simulink model "FLC_PID_Robot_Control_Full"  (R2020b)
settings: Solver=ode4  StartTime=0.0  StopTime=50  FixedStep=0.01  RelTol=1e-3
values from neighbouring files (symbols this model uses):
  a = 0    [Robot_Parameters.m]
  b = 0.2    [Robot_Parameters.m]
  I = 0.08    [Robot_Parameters.m]
  Ke = 0.03    [Robot_Parameters.m]
  Kt = 0.001    [Robot_Parameters.m]
  L = 0.01    [Robot_Parameters.m]
  m = 1.733    [Robot_Parameters.m]
  N = 30    [Robot_Parameters.m]
  r = 0.0425    [Robot_Parameters.m]
  R = 0.7    [Robot_Parameters.m]
libraries: pid_lib x2, fuzblock x1, mobileRoboticsLib x1, simulink x1
settings Model: OrderedModelArguments=off  Creator=dell  LastModifiedBy=dell

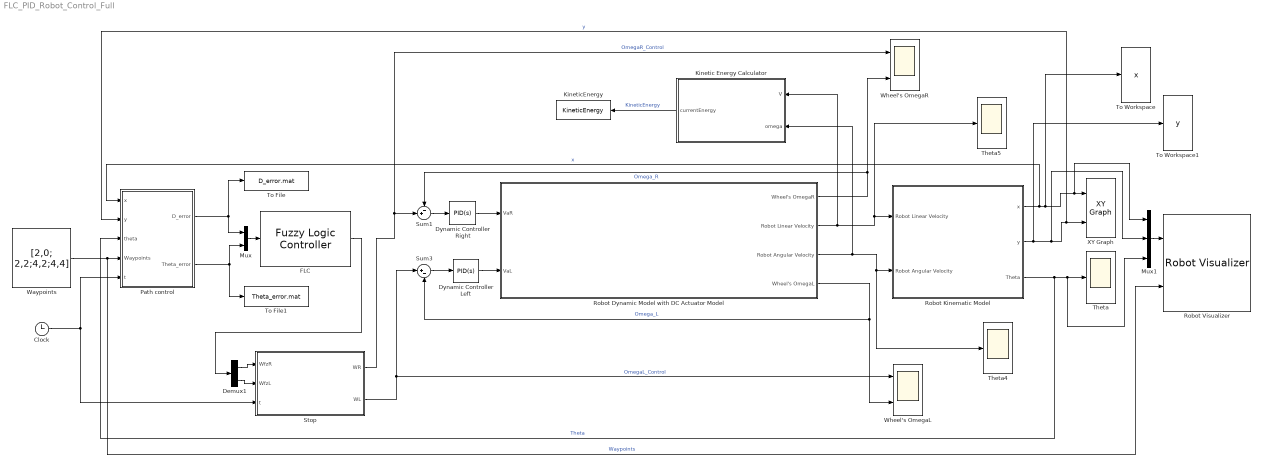
== system FLC_PID_Robot_Control_Full ==
  Clock : Clock
  Demux1 : Demux  Outputs=2
  Dynamic Controller Left : pid_lib/PID Controller  Controller=PID  Form=Parallel  TimeDomain=Continuous-time  UseExternalTs=off  SampleTime=-1  IntegratorMethod=Forward Euler  FilterMethod=Forward Euler  ControllerParametersSource=internal  P=0.75291038869307  I=8.52783510111841  D=-0.0138279489870919  UseFilter=on  N=14.2847240550013  TunerSelectOption=Transfer Function Based (PID Tuner App)  InitialConditionSource=internal  InitialConditionForIntegrator=0  InitialConditionForFilter=0  DifferentiatorICPrevScaledInput=0  ExternalReset=none  TrackingMode=off  Kt=1  LimitOutput=off  SatLimitsSource=internal  UpperSaturationLimit=inf  LowerSaturationLimit=-inf  LinearizeAsGain=on  AntiWindupMode=none  Kb=1  POutMin=[]  POutMax=[]  IOutMin=[]  IOutMax=[]  DOutMin=[]  DOutMax=[]  NOutMin=[]  NOutMax=[]  SumOutMin=[]  SumOutMax=[]  SaturationOutMin=[]  SaturationOutMax=[]  PParamMin=[]  PParamMax=[]  IParamMin=[]  IParamMax=[]  DParamMin=[]  DParamMax=[]  NParamMin=[]  NParamMax=[]  KbParamMin=[]  KbParamMax=[]  KtParamMin=[]  KtParamMax=[]  KbOutMin=[]  KbOutMax=[]  KtOutMin=[]  KtOutMax=[]  IntegratorOutMin=[]  IntegratorOutMax=[]  FilterOutMin=[]  FilterOutMax=[]  SumI1OutMin=[]  SumI1OutMax=[]  SumI2OutMin=[]  SumI2OutMax=[]  SumI3OutMin=[]  SumI3OutMax=[]  SumI4OutMin=[]  SumI4OutMax=[]  SumDOutMin=[]  SumDOutMax=[]  DifferentiatorOutMin=[]  DifferentiatorOutMax=[]  FilterDiffOutCoefMin=[]  FilterDiffOutCoefMax=[]  ReciprocalOutMin=[]  ReciprocalOutMax=[]  SumDenOutMin=[]  SumDenOutMax=[]  SumNumOutMin=[]  SumNumOutMax=[]  DivideOutMin=[]  DivideOutMax=[]  UdiffTsProdOutMin=[]  UdiffTsProdOutMax=[]  NTsProdOutMin=[]  NTsProdOutMax=[]  UintegralTsProdOutMin=[]  UintegralTsProdOutMax=[]  UngainTsProdOutMin=[]  UngainTsProdOutMax=[]  IntegratorContinuousStateAttributes=''  IntegratorStateMustResolveToSignalObject=off  IntegratorRTWStateStorageClass=Auto  FilterContinuousStateAttributes=''  FilterStateMustResolveToSignalObject=off  FilterRTWStateStorageClass=Auto  ParallelPVariant=InternalParameters  IdealPVariant=Disabled  IVariant=InternalParameters  DVariant=InternalParameters  IntegratorVariant=Continuous  SatVariant=Disabled  AWVariant=Passthrough  PCopyVariant=Disabled  TRVariant=Disabled  FdbkBlocksVariant=Forward  IdealPFdbkVariant=Disabled  SatFdbkVariant=Disabled  DerivativeFilterVariant=ContFilter  NVariant=InternalParameters  NCopyVariant=Disabled  FilterICVariant=InternalICsFilter  IntegratorICVariant=InternalICs  ExternalResetVariant=Disabled  TRSumVariant=Passthrough  SumFdbkVariant=Disabled  SumVariant=Sum_PID  TsampFilterVariant=InternalTs  TsampNgainVariant=Passthrough  TsampIntegralVariant=Passthrough  ExternalSaturationOutDataTypeStr=Inherit: Same as second input
  Dynamic Controller Right : pid_lib/PID Controller  Controller=PID  Form=Parallel  TimeDomain=Continuous-time  UseExternalTs=off  SampleTime=-1  IntegratorMethod=Forward Euler  FilterMethod=Forward Euler  ControllerParametersSource=internal  P=0.926055377132756  I=9.27563715391367  D=-0.025  UseFilter=on  N=20.0890041410903  TunerSelectOption=Transfer Function Based (PID Tuner App)  ZeroCross=off  InitialConditionSource=internal  InitialConditionForIntegrator=0  InitialConditionForFilter=0  DifferentiatorICPrevScaledInput=0  ExternalReset=none  TrackingMode=off  Kt=1  LimitOutput=off  SatLimitsSource=internal  UpperSaturationLimit=inf  LowerSaturationLimit=-inf  LinearizeAsGain=on  AntiWindupMode=none  Kb=1  POutMin=[]  POutMax=[]  IOutMin=[]  IOutMax=[]  DOutMin=[]  DOutMax=[]  NOutMin=[]  NOutMax=[]  SumOutMin=[]  SumOutMax=[]  SaturationOutMin=[]  SaturationOutMax=[]  PParamMin=[]  PParamMax=[]  IParamMin=[]  IParamMax=[]  DParamMin=[]  DParamMax=[]  NParamMin=[]  NParamMax=[]  KbParamMin=[]  KbParamMax=[]  KtParamMin=[]  KtParamMax=[]  KbOutMin=[]  KbOutMax=[]  KtOutMin=[]  KtOutMax=[]  IntegratorOutMin=[]  IntegratorOutMax=[]  FilterOutMin=[]  FilterOutMax=[]  SumI1OutMin=[]  SumI1OutMax=[]  SumI2OutMin=[]  SumI2OutMax=[]  SumI3OutMin=[]  SumI3OutMax=[]  SumI4OutMin=[]  SumI4OutMax=[]  SumDOutMin=[]  SumDOutMax=[]  DifferentiatorOutMin=[]  DifferentiatorOutMax=[]  FilterDiffOutCoefMin=[]  FilterDiffOutCoefMax=[]  ReciprocalOutMin=[]  ReciprocalOutMax=[]  SumDenOutMin=[]  SumDenOutMax=[]  SumNumOutMin=[]  SumNumOutMax=[]  DivideOutMin=[]  DivideOutMax=[]  UdiffTsProdOutMin=[]  UdiffTsProdOutMax=[]  NTsProdOutMin=[]  NTsProdOutMax=[]  UintegralTsProdOutMin=[]  UintegralTsProdOutMax=[]  UngainTsProdOutMin=[]  UngainTsProdOutMax=[]  IntegratorContinuousStateAttributes=''  IntegratorStateMustResolveToSignalObject=off  IntegratorRTWStateStorageClass=Auto  FilterContinuousStateAttributes=''  FilterStateMustResolveToSignalObject=off  FilterRTWStateStorageClass=Auto  ParallelPVariant=InternalParameters  IdealPVariant=Disabled  IVariant=InternalParameters  DVariant=InternalParameters  IntegratorVariant=Continuous  SatVariant=Disabled  AWVariant=Passthrough  PCopyVariant=Disabled  TRVariant=Disabled  FdbkBlocksVariant=Forward  IdealPFdbkVariant=Disabled  SatFdbkVariant=Disabled  DerivativeFilterVariant=ContFilter  NVariant=InternalParameters  NCopyVariant=Disabled  FilterICVariant=InternalICsFilter  IntegratorICVariant=InternalICs  ExternalResetVariant=Disabled  TRSumVariant=Passthrough  SumFdbkVariant=Disabled  SumVariant=Sum_PID  TsampFilterVariant=InternalTs  TsampNgainVariant=Passthrough  TsampIntegralVariant=Passthrough  ExternalSaturationOutDataTypeStr=Inherit: Same as second input
  FLC : fuzblock/Fuzzy Logic  Controller  FIS="\"D:\\PhDDATA\\PhDBrno\\Final_Dissertation\\Experiment\\SoftWare_Hardwares\\FLC_PID_Robot_Control_Full\\FuzzyLogicControllers_FIS\\Proposed_GA_FLC.fis\""  OutputSampleNumber=101  DataType=double  FuzzifiedInputs=off  RuleFiringStrengths=off  RuleOutputs=off  AggregatedOutputs=off  SimulateUsing=Interpreted execution  OutOfRangeInputValueMessage=warning  NoRuleFiredMessage=warning  EmptyOutputFuzzySetMessage=warning
  Kinetic Energy Calculator : MATLAB Function  TreatAsAtomicUnit=on
  KineticEnergy : ToWorkspace  VariableName=KineticEnergy  SaveFormat=Timeseries  SampleTime=-1
  Mux : Mux  Inputs=2
  Mux1 : Mux  Inputs=3
  Path control : MATLAB Function  TreatAsAtomicUnit=on
  Robot Dynamic Model with DC Actuator Model : Subsystem
  Robot Kinematic Model : Subsystem
  Robot Visualizer : mobileRoboticsLib/Environments/Robot Visualizer  Priority=99  robotRadius=0.0425  showTrajectory=on  hasWaypoints=on  hasLidar=off  sensorOffset=[ 0 0 ]  scanAngles=0  hasObjDetector=off  objDetectorOffset=[ 0, 0 ]  objDetectorAngle=0  objDetectorFOV=0  objDetectorMaxRange=0  objectColors=0  objectMarkers=s
      settings: SourceProductName=Ground Vehicles Library
  Stop : MATLAB Function  TreatAsAtomicUnit=on
  Sum1 : Sum  Inputs=-+|
  Sum3 : Sum  Inputs=|+-
  Theta : Scope
  Theta4 : Scope
  Theta5 : Scope
  To File : ToFile  Filename=D_error.mat  SaveFormat=Timeseries
  To File1 : ToFile  Filename=Theta_error.mat  SaveFormat=Timeseries
  To Workspace : ToWorkspace  VariableName=x  SaveFormat=Timeseries  SampleTime=-1
  To Workspace1 : ToWorkspace  VariableName=y  SaveFormat=Timeseries  SampleTime=-1
  Waypoints : Constant  Value=[2,0; 2,2;4,2;4,4]  SampleTime=-1
  Wheel's OmegaL : Scope  NumInputPorts=2
  Wheel's OmegaR : Scope  NumInputPorts=2
  XY Graph : simulink/Sinks/XY Graph  xmin=-2.5  xmax=6  ymin=-0.5  ymax=6  st=-1
  wires:
  Sum1/1 -> Dynamic Controller Right/1
  Sum3/1 -> Dynamic Controller Left/1
  Robot Kinematic Model/1(x) -> To Workspace/1, XY Graph/1, Mux1/1, Path control/1(x)  "x"
  Robot Kinematic Model/2(y) -> To Workspace1/1, XY Graph/2, Path control/2(y), Mux1/2  "y"
  Robot Kinematic Model/3(Theta) -> Theta/1, Mux1/3, Path control/3(theta)  "Theta"
  Robot Dynamic Model with DC Actuator Model/2(Robot Linear Velocity) -> Robot Kinematic Model/1(Robot Linear Velocity), Theta5/1, Kinetic Energy Calculator/1(V)
  Dynamic Controller Right/1 -> Robot Dynamic Model with DC Actuator Model/1(VaR)
  Dynamic Controller Left/1 -> Robot Dynamic Model with DC Actuator Model/2(VaL)
  Robot Dynamic Model with DC Actuator Model/4(Wheel's OmegaL) -> Sum3/2, Wheel's OmegaL/2  "Omega_L"
  Stop/1(WR) -> Wheel's OmegaR/1, Sum1/2  "OmegaR_Control"
  Stop/2(WL) -> Sum3/1, Wheel's OmegaL/1  "OmegaL_Control"
  Mux/1 -> FLC/1
  Path control/1(D_error) -> Mux/1, To File/1
  Path control/2(Theta_error) -> Mux/2, To File1/1
  Waypoints/1 -> Robot Visualizer/2, Path control/4(Waypoints)  "Waypoints"
  Mux1/1 -> Robot Visualizer/1
  Robot Dynamic Model with DC Actuator Model/1(Wheel's OmegaR) -> Wheel's OmegaR/2, Sum1/1  "Omega_R"
  Kinetic Energy Calculator/1(currentEnergy) -> KineticEnergy/1  "KineticEnergy"
  Robot Dynamic Model with DC Actuator Model/3(Robot Angular Velocity) -> Robot Kinematic Model/2(Robot Angular Velocity), Theta4/1, Kinetic Energy Calculator/2(omega)
  Demux1/1 -> Stop/1(WfzR)
  Demux1/2 -> Stop/2(WfzL)
  FLC/1 -> Demux1/1
  Clock/1 -> Path control/5(t), Stop/3(t)

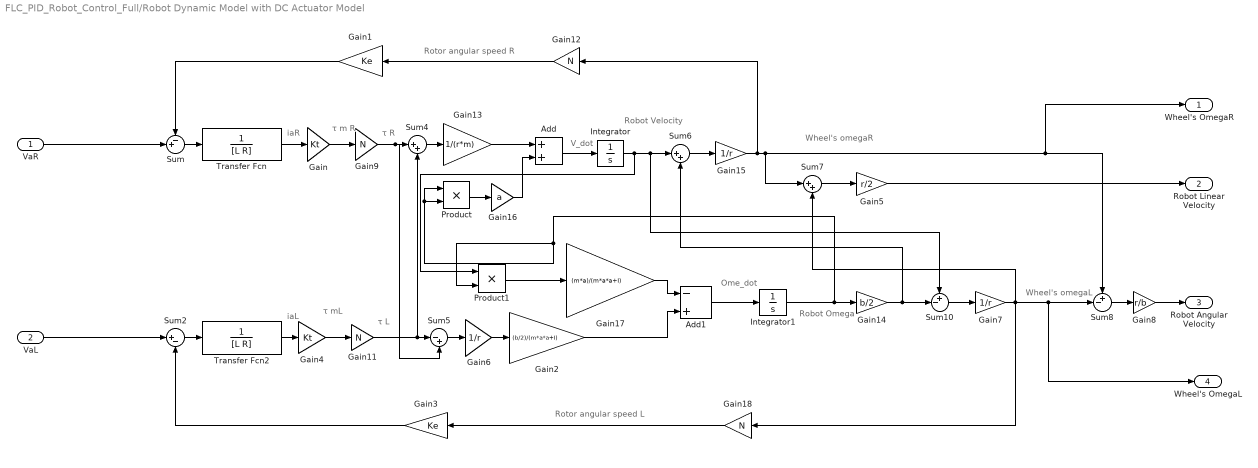
== system FLC_PID_Robot_Control_Full/Robot Dynamic Model with DC Actuator Model ==
  note: Rotor angular speed R
  note: Robot Velocity
  note: V_dot
  note: Robot Omega
  note: Ome_dot
  note: τ R
  note: τ m R
  note: iaR
  note: iaL
  note: τ mL
  note: τ L
  note: Rotor angular speed L
  note: Wheel's omegaR
  note: Wheel's omegaL
  VaR : Inport
  VaL : Inport  Port=2
  Add : Sum
  Add1 : Sum  Inputs=-+
  Gain : Gain  Gain=Kt
  Gain1 : Gain  Gain=Ke
  Gain{9,11..12,18} (4 alike) : Gain  Gain=N
  Gain13 : Gain  Gain=1/(r*m)
  Gain14 : Gain  Gain=b/2
  Gain15 : Gain  Gain=1/r
  Gain16 : Gain  Gain=a
  Gain17 : Gain  Gain=(m*a)/(m*a*a+I)
  Gain2 : Gain  Gain=(b/2)/(m*a*a+I)
  Gain3 : Gain  Gain=Ke
  Gain4 : Gain  Gain=Kt
  Gain5 : Gain  Gain=r/2
  Gain6 : Gain  Gain=1/r
  Gain7 : Gain  Gain=1/r
  Gain8 : Gain  Gain=r/b
  Integrator : Integrator
  Integrator1 : Integrator
  Product : Product
  Product1 : Product
  Sum : Sum  Inputs=-+|
  Sum10 : Sum  Inputs=+-|
  Sum2 : Sum  Inputs=|+-
  Sum4 : Sum  Inputs=|++
  Sum5 : Sum  Inputs=|-+
  Sum6 : Sum  Inputs=|++
  Sum7 : Sum  Inputs=|++
  Sum8 : Sum  Inputs=+-|
  Transfer Fcn : TransferFcn  Denominator=[L R]
  Transfer Fcn2 : TransferFcn  Denominator=[L R]
  Wheel's OmegaR : Outport
  Robot Linear Velocity : Outport  Port=2
  Robot Angular Velocity : Outport  Port=3
  Wheel's OmegaL : Outport  Port=4
  wires:
  Gain8/1 -> Robot Angular Velocity/1
  Gain5/1 -> Robot Linear Velocity/1
  Integrator/1 -> Sum6/1, Sum10/1, Product1/1
  Gain2/1 -> Add1/2
  Gain4/1 -> Gain11/1
  Sum6/1 -> Gain15/1
  Gain14/1 -> Sum10/2, Sum6/2
  Gain1/1 -> Sum/1
  Gain15/1 -> Gain12/1, Wheel's OmegaR/1, Sum8/1, Sum7/1
  Sum7/1 -> Gain5/1
  Gain6/1 -> Gain2/1
  Integrator1/1 -> Gain14/1, Product/2, Product/1, Product1/2
  Sum10/1 -> Gain7/1
  Product1/1 -> Gain17/1
  Transfer Fcn2/1 -> Gain4/1
  Sum/1 -> Transfer Fcn/1
  Gain17/1 -> Add1/1
  Add/1 -> Integrator/1
  Add1/1 -> Integrator1/1
  Gain12/1 -> Gain1/1
  Gain7/1 -> Wheel's OmegaL/1, Sum8/2, Sum7/2, Gain18/1
  Product/1 -> Gain16/1
  Gain9/1 -> Sum4/1, Sum5/2
  Gain/1 -> Gain9/1
  Gain11/1 -> Sum5/1, Sum4/2
  Gain16/1 -> Add/2
  Sum8/1 -> Gain8/1
  Gain18/1 -> Gain3/1
  Sum2/1 -> Transfer Fcn2/1
  Gain3/1 -> Sum2/2
  VaL/1 -> Sum2/1
  Transfer Fcn/1 -> Gain/1
  Gain13/1 -> Add/1
  Sum4/1 -> Gain13/1
  Sum5/1 -> Gain6/1
  VaR/1 -> Sum/2

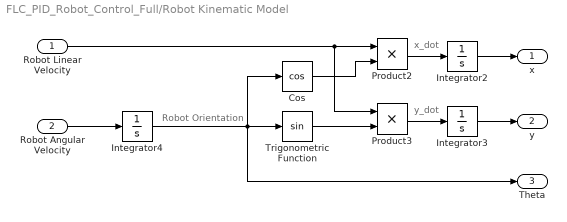
== system FLC_PID_Robot_Control_Full/Robot Kinematic Model ==
  note: x_dot
  note: Robot Orientation
  note: y_dot
  Robot Linear Velocity : Inport
  Robot Angular Velocity : Inport  Port=2
  Cos : Trigonometry  Operator=cos
  Integrator2 : Integrator
  Integrator3 : Integrator
  Integrator4 : Integrator
  Product2 : Product
  Product3 : Product
  Trigonometric Function : Trigonometry
  x : Outport
  y : Outport  Port=2
  Theta : Outport  Port=3
  wires:
  Trigonometric Function/1 -> Product3/2
  Cos/1 -> Product2/2
  Robot Linear Velocity/1 -> Product2/1, Product3/1
  Integrator4/1 -> Cos/1, Theta/1, Trigonometric Function/1
  Integrator2/1 -> x/1
  Product3/1 -> Integrator3/1
  Product2/1 -> Integrator2/1
  Integrator3/1 -> y/1
  Robot Angular Velocity/1 -> Integrator4/1

== matlab function FLC_PID_Robot_Control_Full/Path control ==
  data: x input; y input; theta input; D_error output; Theta_error output; Waypoints input; t input
%----------------------------------------------------------------------------------------------
%--------------------------------------------------------------------------------------------
function [D_error, Theta_error] = fcn(x,y,theta,Waypoints,t)
%  Go to the Waypoint 1
Pi = 3.14;
distanceEps = 0.01;
x_w = Waypoints(1,1);
y_w = Waypoints(1,2);
deltaX = x_w - x;
deltaY = y_w - y;
D_error = sqrt(deltaX^2 + deltaY^2);
Theta_w = atan2(deltaY,deltaX);
Theta_error = Theta_w - theta;
if Theta_error > Pi
    Theta_error = Theta_error - 2*Pi;
end
if Theta_error < -Pi
    Theta_error = Theta_error + 2*Pi;
end 
%  Go to the Waypoint 2
if D_error < distanceEps
    i = 2;
    x_w = Waypoints(i,1);
    y_w = Waypoints(i,2);
    deltaX = x_w - x;
    deltaY = y_w - y;
    D_error = sqrt(deltaX^2 + deltaY^2)
    Theta_w = atan2(deltaY,deltaX);
    Theta_error = Theta_w - theta;
    if Theta_error > Pi
        Theta_error = Theta_error- 2*Pi;
    end
    if Theta_error < -Pi
        Theta_error = Theta_error + 2*Pi;
    end
elseif (D_error >= distanceEps) && (t >= 5.31)
    i = 2;
    x_w = Waypoints(i,1);
    y_w = Waypoints(i,2);
    deltaX = x_w - x;
    deltaY = y_w - y;
    D_error = sqrt(deltaX^2 + deltaY^2)
    Theta_w = atan2(deltaY,deltaX);
    Theta_error = Theta_w - theta;
    if Theta_error > Pi
        Theta_error = Theta_error- 2*Pi;
    end
    if Theta_error < -Pi
        Theta_error = Theta_error + 2*Pi;
    end
    %  Go to the Waypoint 3
    if D_error < distanceEps
        i = 3;
        x_w = Waypoints(i,1);
        y_w = Waypoints(i,2);
        deltaX = x_w - x;
        deltaY = y_w - y;
        D_error = sqrt(deltaX^2 + deltaY^2)
        Theta_w = atan2(deltaY,deltaX);
        Theta_error = Theta_w - theta;
        if Theta_error > Pi
            Theta_error = Theta_error- 2*Pi;
        end
        if Theta_error < -Pi
            Theta_error = Theta_error + 2*Pi;
        end
    elseif (D_error >= distanceEps) && (t >= 10.9)
        i = 3;
        x_w = Waypoints(i,1);
        y_w = Waypoints(i,2);
        deltaX = x_w - x;
        deltaY = y_w - y;
        D_error = sqrt(deltaX^2 + deltaY^2)
        Theta_w = atan2(deltaY,deltaX);
        Theta_error = Theta_w - theta;
        if Theta_error > Pi
            Theta_error = Theta_error- 2*Pi;
        end
        if Theta_error < -Pi
            Theta_error = Theta_error + 2*Pi;
        end
        %  Go to the Waypoint 4 (GOAL)
        if D_error < distanceEps
            i = 4;
            x_w = Waypoints(i,1);
            y_w = Waypoints(i,2);
            deltaX = x_w - x;
            deltaY = y_w - y;
            D_error = sqrt(deltaX^2 + deltaY^2)
            Theta_w = atan2(deltaY,deltaX);
            Theta_error = Theta_w - theta;
            if Theta_error > Pi
                Theta_error = Theta_error- 2*Pi;
            end
            if Theta_error < -Pi
                Theta_error = Theta_error + 2*Pi;
            end
        elseif (D_error >= distanceEps) && (t >= 17.2)
            i = 4;
            x_w = Waypoints(i,1);
            y_w = Waypoints(i,2);
            deltaX = x_w - x;
            deltaY = y_w - y;
            D_error = sqrt(deltaX^2 + deltaY^2)
            Theta_w = atan2(deltaY,deltaX);
            Theta_error = Theta_w - theta;
            if Theta_error > Pi
                Theta_error = Theta_error- 2*Pi;
            end
            if Theta_error < -Pi
                Theta_error = Theta_error + 2*Pi;
            end            
        end
    end
end
%--------------------------------------------------------------------------------------------
%--------------------------------------------------------------------------------------------

== matlab function FLC_PID_Robot_Control_Full/Stop ==
  data: WfzR input; WfzL input; WR output; WL output; t input
function [WR,WL] = fcn(WfzR,WfzL,t)   
    WR = WfzR;
    WL = WfzL;    
if t >= 22.8
    WR = 0;
    WL = 0;
end    
end

== matlab function FLC_PID_Robot_Control_Full/Kinetic Energy Calculator ==
  data: V input; omega input; currentEnergy output
function currentEnergy    = fcn(V,omega)
m = 1.733;
I = 0.08;
currentEnergy = 0.5*(m*V*V + I*omega*omega);
end
